simulink model "parallelizationTest"  (R2017a)
settings: Solver=FixedStepAuto  StartTime=0.0  StopTime=Inf  FixedStep=0.1  RelTol=1e-3
settings Model: Creator=TSu  LastModifiedBy=TSu
settings SolverCC: AutoInsertRateTranBlk=on
settings DebuggingCC: RootOutportRequireBusObject=error  StrictBusMsg=ErrorOnBusTreatedAsVector
settings HardwareCC: ProdBitPerLong=64  ProdBitPerPointer=32  ProdBitPerSizeT=32  ProdBitPerPtrDiffT=32  ProdLargestAtomicFloat=None  ProdHWDeviceType=Generic->Custom
settings RTWCC: SystemTargetFile=NIVeriStand_Linux_64.tlc  GenCodeOnly=on  PackageGeneratedCodeAndArtifacts=on  PackageName=parallelTest  TemplateMakefile=NIVeriStand_Linux_64.tmf  Description=NI Linux Real-Time (64-bit) Target
settings STFCustomTargetCC: TargetLangStandard=C99 (ISO)  MatFileLogging=on  MATLABClassNameForMDSCustomization=Simulink.SoftwareTarget.TargetSpecificTriggerConfigurationBase  SystemTargetFile=NIVeriStand_Linux_64.tlc

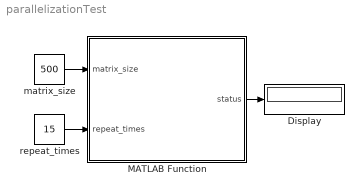
== system parallelizationTest ==
  Display : Display
      settings: Decimation=2
  MATLAB Function : MATLAB Function  TreatAsAtomicUnit=on
  matrix_size : Constant  Value=500
  repeat_times : Constant  Value=15
  wires:
  matrix_size/1 -> MATLAB Function/1(matrix_size)
  repeat_times/1 -> MATLAB Function/2(repeat_times)
  MATLAB Function/1(status) -> Display/1

== matlab function parallelizationTest/MATLAB Function ==
  data: matrix_size input; status output; repeat_times input
function status = time_par_tests(matrix_size, repeat_times)
% time_par_tests: Perform a parallization test (baseline)

%status = time_par_tests_mfile(matrix_size, repeat_times);

M = repeat_times; %[-] how many times we repeat the operation
N = matrix_size; %[-] matrix size

seed = 42; % Specify the seed for MATLAB random number generator
rng(seed);

a = zeros(1,M); %[-] soring the results
parfor i = 1:M
    a(i) = max(abs(eig(rand(N))));
end

status = 0;

end
